simulink model "class_3_simulink"  (R2023b)
settings: Solver=VariableStepAuto  StartTime=0.0  StopTime=25  RelTol=1e-3
values from neighbouring files (symbols this model uses):
  denp = [3 1]    [class_3.m]
  h = 6.5    [class_3.m]
  I = eye(size(A))    [class_3.m]
  K = 6.7*(-A)    [class_3.m]
  kr = (c*((B*K-A)^(-1))*B)^(-1)    [class_3.m]
  nump = [0 2]    [class_3.m]
  s = tf('s')    [class_3.m]
undefined symbols (not defined in the file or in its folder): A, B
libraries: cstblocks x6
settings Model: Creator=klysm  LastModifiedBy=klysm

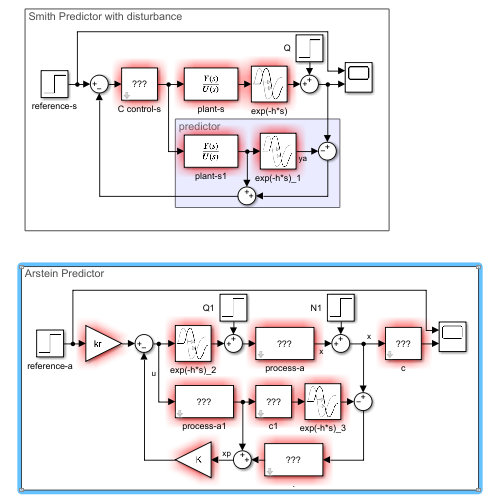
[thumbnail: Simulink's stored preview of the top-level diagram]
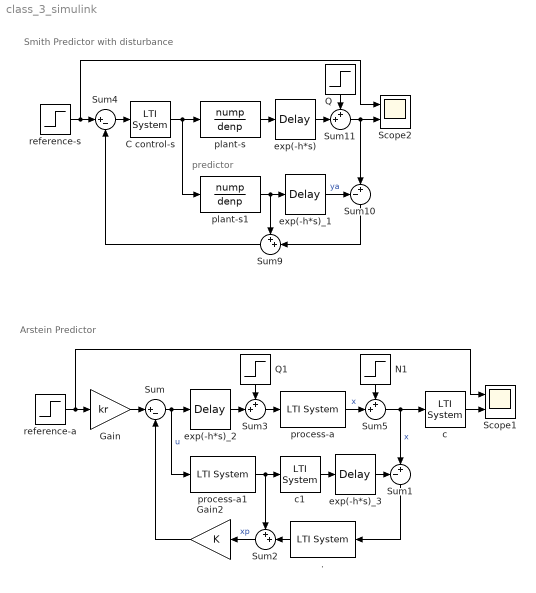
== system class_3_simulink ==
  note: Arstein Predictor
  note: Smith Predictor with disturbance
  note: predictor
  . : cstblocks/LTI System  sys=exp(A*h)  IC=[]  PadeOrder=0
  C control-s : cstblocks/LTI System  sys=C  IC=[]  PadeOrder=0
  Gain : Gain  Gain=kr
  Gain2 : Gain  Gain=K
  N1 : Step  Time=25  After=0.2  SampleTime=0
  Q : Step  Time=12  After=0.2  SampleTime=0
  Q1 : Step  Time=12  After=0.2  SampleTime=0
  Scope1 : Scope  NumInputPorts=2
  Scope2 : Scope  NumInputPorts=2
  Sum : Sum  Inputs=|+-
  Sum1 : Sum  Inputs=-+|
  Sum10 : Sum  Inputs=-+|
  Sum{2..3,5,9,11} (5 alike) : Sum  Inputs=++|
  Sum4 : Sum  Inputs=|+-
  c : cstblocks/LTI System  sys=c  IC=[]  PadeOrder=0
  c1 : cstblocks/LTI System  sys=c  IC=[]  PadeOrder=0
  exp(-h*s) : TransportDelay  DelayTime=h
  exp(-h*s)_1 : TransportDelay  DelayTime=h
  exp(-h*s)_2 : TransportDelay  DelayTime=h
  exp(-h*s)_3 : TransportDelay  DelayTime=h
  plant-s : TransferFcn  Numerator=nump  Denominator=denp
  plant-s1 : TransferFcn  Numerator=nump  Denominator=denp
  process-a : cstblocks/LTI System  sys=inv(s*I-A)*B  IC=[]  PadeOrder=0
  process-a1 : cstblocks/LTI System  sys=inv(s*I-A)*B  IC=[]  PadeOrder=0
  reference-a : Step  Time=0  SampleTime=0
  reference-s : Step  Time=0  SampleTime=0
  wires:
  Gain/1 -> Sum/1
  reference-a/1 -> Scope1/1, Gain/1
  Sum/1 -> process-a1/1, exp(-h*s)_2/1  "u"
  exp(-h*s)_2/1 -> Sum3/2
  process-a1/1 -> c1/1, Sum2/1
  Sum5/1 -> c/1, Sum1/2  "x"
  exp(-h*s)_3/1 -> Sum1/1
  ./1 -> Sum2/2
  Sum1/1 -> ./1
  Sum2/1 -> Gain2/1  "xp"
  Gain2/1 -> Sum/2
  Sum3/1 -> process-a/1
  Q1/1 -> Sum3/1
  Sum4/1 -> C control-s/1
  C control-s/1 -> plant-s/1, plant-s1/1
  plant-s/1 -> exp(-h*s)/1
  reference-s/1 -> Scope2/1, Sum4/1
  plant-s1/1 -> Sum9/1, exp(-h*s)_1/1
  exp(-h*s)_1/1 -> Sum10/1  "ya"
  Q/1 -> Sum11/1
  Sum10/1 -> Sum9/2
  Sum11/1 -> Sum10/2, Scope2/2
  Sum9/1 -> Sum4/2
  exp(-h*s)/1 -> Sum11/2
  c/1 -> Scope1/2
  c1/1 -> exp(-h*s)_3/1
  process-a/1 -> Sum5/2  "x"
  N1/1 -> Sum5/1
